simulink library "MFMdl4_new"  (Simulink 8.8)
settings: Solver=VariableStepAuto  StartTime=0.0  StopTime=10.0  RelTol=1e-3
libraries: simulink x2
settings Model: Creator=viett  LastModifiedBy=hahoa

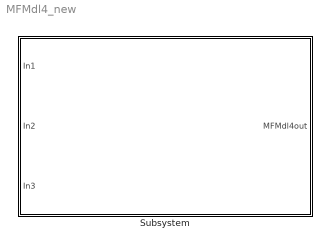
== system MFMdl4_new ==
  Subsystem : Subsystem

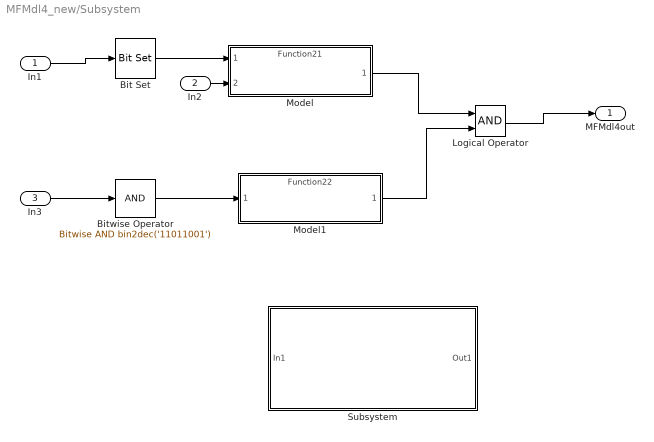
== system MFMdl4_new/Subsystem ==
  In1 : Inport
  In2 : Inport  Port=2
  In3 : Inport  Port=3
  Bit Set : simulink/Logic and Bit Operations/Bit Set  iBit=0
  Bitwise Operator : simulink/Logic and Bit Operations/Bitwise Operator  logicop=AND  UseBitMask=on  BitMask=bin2dec('11011001')  BitMaskRealWorld=Stored Integer
  Logical Operator : Logic  AllPortsSameDT=off  OutDataTypeStr=boolean
  Model : ModelReference  ModelNameDialog=Function21.slx  SimulationMode=Normal  ModelReferenceVersion=1.3
  Model1 : ModelReference  ModelNameDialog=Function22.slx  SimulationMode=Normal  ModelReferenceVersion=1.3
  Subsystem : Subsystem
  MFMdl4out : Outport
  wires:
  Model1/1 -> Logical Operator/2
  Bitwise Operator/1 -> Model1/1
  Model/1 -> Logical Operator/1
  Bit Set/1 -> Model/1
  In2/1 -> Model/2
  In3/1 -> Bitwise Operator/1
  In1/1 -> Bit Set/1
  Logical Operator/1 -> MFMdl4out/1

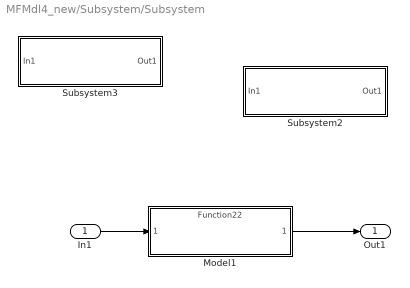
== system MFMdl4_new/Subsystem/Subsystem ==
  In1 : Inport
  Model1 : ModelReference  ModelNameDialog=Function22.slx  SimulationMode=Normal  ModelReferenceVersion=1.3
  Subsystem2 : Subsystem
  Subsystem3 : Subsystem
  Out1 : Outport
  wires:
  In1/1 -> Model1/1
  Model1/1 -> Out1/1

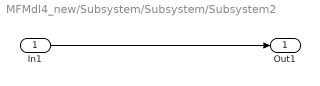
== system MFMdl4_new/Subsystem/Subsystem/Subsystem2 ==
  In1 : Inport
  Out1 : Outport
  wires:
  In1/1 -> Out1/1

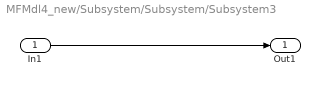
== system MFMdl4_new/Subsystem/Subsystem/Subsystem3 ==
  In1 : Inport
  Out1 : Outport
  wires:
  In1/1 -> Out1/1
